simulink model "malha_aberta_simu"  (R2018a)
settings: Solver=VariableStepAuto  StartTime=0.0  StopTime=11.0  RelTol=1e-3
values from neighbouring files (symbols this model uses):
  Km = 460    [LineFollower.m]    (also in malha_aberta.m = 455.5; malha_fechada.m = 455.5)
  Pm = 12.97    [LineFollower.m]    (also in malha_aberta.m; malha_fechada.m)
  Ts = 1e-3    (= 0.001)    [LineFollower.m]    (also in Untitled.m; calculo_erros.m; ft_speedw.mat; malha_aberta.m)
settings Model: Creator=bruno  LastModifiedBy=bruno

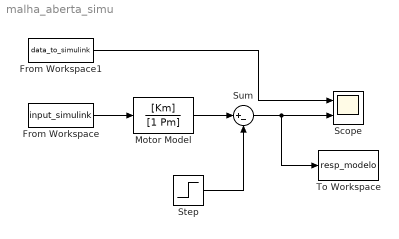
== system malha_aberta_simu ==
  From Workspace : FromWorkspace  VariableName=input_simulink  SampleTime=Ts
  From Workspace1 : FromWorkspace  VariableName=data_to_simulink  SampleTime=Ts
  Motor Model : TransferFcn  Numerator=[Km]  Denominator=[1 Pm]
  Scope : Scope  NumInputPorts=2
  Step : Step  After=160  SampleTime=Ts
  Sum : Sum  Inputs=|+-
  To Workspace : ToWorkspace  VariableName=resp_modelo  SampleTime=Ts
      settings: Save2DSignal=2-D array (concatenate along first dimension)
  wires:
  From Workspace/1 -> Motor Model/1
  From Workspace1/1 -> Scope/1
  Motor Model/1 -> Sum/1
  Sum/1 -> To Workspace/1, Scope/2
  Step/1 -> Sum/2
